simulink model "boostr"  (Simulink 10.0)
settings: Solver=ode23tb  StartTime=0.0  StopTime=1  MaxStep=1e-6  RelTol=1e-3  EnableMultiTasking=on
undefined symbols (not defined in the file): C, D, fs, L, R, Vin1
libraries: powerlib x10
settings Model: Creator=UDHAYA KUMAR  LastModifiedBy=bhisma
settings SolverCC: ZeroCrossControl=DisableAll  AutoInsertRateTranBlk=on
settings DataIOCC: LimitDataPoints=on  SignalLoggingSaveFormat=ModelDataLogs
settings OptimizationCC: ExpressionDepthLimit=2147483647
settings DebuggingCC: FcnCallInpInsideContextMsg=warning  StateNameClashWarn=warning
settings GRTTargetCC: GeneratePreprocessorConditionals=Disable all
settings ConfigComp: CovExternalEMLEnable=off

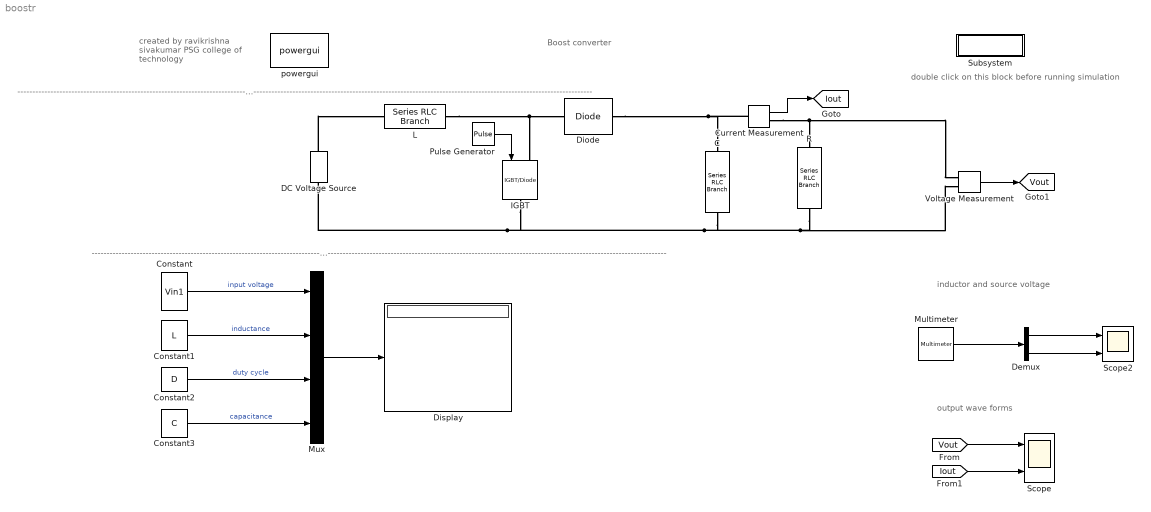
== system boostr ==
  note: Boost converter
  note: inductor and source voltage
  note: created by
      | ravikrishna sivakumar
      | PSG college of technology
  note: output wave forms
  note: double click on this block before running simulation
  note: --------------------------------------------------------------------------------------------------------------------------------------------------------------------------------------------------------------------------------------------------
  note: ---------------------------------------------------------------------------------------------------------------------------------------------------------------------------------------------------------------------------------------------------
  C : powerlib/Elements/Series RLC Branch  PhysicalDomain=powersysdomain  SubClassName=unknown  LeftPortType=p1  RightPortType=p1  LConnTagsString=__new0  RConnTagsString=__new0  BranchType=C  Resistance=1  Inductance=1e-3  SetiL0=off  InitialCurrent=0  Capacitance=C  Setx0=off  InitialVoltage=0  Measurements=None
      settings: SourceProductName=Simscape Electrical
  Constant : Constant  Value=Vin1
  Constant1 : Constant  Value=L
  Constant2 : Constant  Value=D
  Constant3 : Constant  Value=C
  Current Measurement : powerlib/Measurements/Current Measurement  SystemSampleTime=-1  PhasorSimulation=off  OutputType=Complex  PSBequivalent=0
      settings: SourceProductName=Simscape Electrical
  DC Voltage Source : powerlib/Electrical Sources/DC Voltage Source  SystemSampleTime=-1  Amplitude=Vin1  Measurements=Voltage
      settings: AttributesFormatString=%<Amplitude>  SourceProductName=Simscape Electrical
  Demux : Demux  Outputs=2
  Diode : powerlib/Power Electronics/Diode  SystemSampleTime=-1  Ron=0.001  Lon=0  Vf=0.8  IC=0  UseSnubber=off  Rs=inf  Cs=0  Measurements=off
      settings: SourceProductName=Simscape Electrical
  Display : Display
  IGBT : powerlib/Power Electronics/IGBT//Diode  SystemSampleTime=-1  Ron=1e-3  Rs=1e5  Cs=inf  Measurements=off
      settings: SourceProductName=Simscape Electrical
  L : powerlib/Elements/Series RLC Branch  PhysicalDomain=powersysdomain  SubClassName=unknown  LeftPortType=p1  RightPortType=p1  LConnTagsString=__new0  RConnTagsString=__new0  BranchType=L  Resistance=1  Inductance=L  SetiL0=on  InitialCurrent=0  Capacitance=1e-6  Setx0=off  InitialVoltage=0  Measurements=Branch voltage
      settings: SourceProductName=Simscape Electrical
  Multimeter : powerlib/Measurements/Multimeter  SystemSampleTime=-1  PhasorSimulation=off  OutputType=Complex  sel=[1 2]  L=2  Gain=[1 1]  yselected={'Ub: L','Usrc: DC Voltage Source'};  PSBOutputType=1  PSBequivalent=0  AxesSetting=[0,0.1,-100,100]  Display=0  SavedBlockNames=-11
      settings: SourceProductName=Simscape Electrical
  Mux : Mux
  Pulse Generator : DiscretePulseGenerator  PulseType=Time based  Period=1/fs  PulseWidth=D
  R : powerlib/Elements/Series RLC Branch  PhysicalDomain=powersysdomain  SubClassName=unknown  LeftPortType=p1  RightPortType=p1  LConnTagsString=__new0  RConnTagsString=__new0  BranchType=R  Resistance=R  Inductance=1e-3  SetiL0=off  InitialCurrent=0  Capacitance=1e-6  Setx0=off  InitialVoltage=0  Measurements=None
      settings: SourceProductName=Simscape Electrical
  Scope : Scope  NumInputPorts=2
  Scope2 : Scope  NumInputPorts=2
  Subsystem : Subsystem
      settings: OpenFcn=open('boost.m')
      mask Display: fprintf('boost')
  Voltage Measurement : powerlib/Measurements/Voltage Measurement  SystemSampleTime=-1  PhasorSimulation=off  OutputType=Complex  PSBequivalent=0
      settings: SourceProductName=Simscape Electrical
  powergui : powerlib/powergui  Priority=1  SystemSampleTime=-1  SimulationMode=Continuous  SampleTime=50e-6  frequency=60  SPID=off  DisableSnubberDevices=off  DisableRonSwitches=off  DisableVfSwitches=off  SwTol=0  Interpol=off  DisplayEquations=off  FunctionMessages=off  frequencyindice=0  Pbase=100e6  ErrMax=1e-4  Iterations=50  UnitsV=kV  UnitsW=MW  echomessages=off  HookPort=off  EnableUseOfTLC=off  x0status=blocks  RestoreLinks=warning  ResistiveCurrentMeasurement=off  Ylog=off  Xlog=on  ShowGrid=off  save=off  variable=ZData  ZoomFFT=off  StartTime=0.0  cycles=1  DisplayStyle=1  FreqAxis=off  MaxFrequency=1000  frequencyindicesteady=1  display=off  methode=off
      settings: SourceProductName=Simscape Electrical
  tag scope: Iout=global, Vout=global
  wires:
  Pulse Generator/1 -> IGBT/1
  Multimeter/1 -> Demux/1
  Demux/1 -> Scope2/1
  Demux/2 -> Scope2/2
  Current Measurement/1 -> [Iout]
  Voltage Measurement/1 -> [Vout]
  [Vout] -> Scope/1
  [Iout] -> Scope/2
  Constant/1 -> Mux/1  "input voltage"
  Constant1/1 -> Mux/2  "inductance"
  Constant2/1 -> Mux/3  "duty cycle"
  Constant3/1 -> Mux/4  "capacitance"
  Mux/1 -> Display/1
  connections:
  Current Measurement/RConn1 -- R/LConn1 -- Voltage Measurement/LConn1
  L/RConn1 -- Diode/LConn1 -- IGBT/LConn1
  R/RConn1 -- C/RConn1 -- DC Voltage Source/LConn1 -- IGBT/RConn1 -- Voltage Measurement/LConn2
  DC Voltage Source/RConn1 -- L/LConn1
  Diode/RConn1 -- C/LConn1 -- Current Measurement/LConn1

== system boostr/Subsystem ==
